simulink model "chap1_1sim"  (Simulink 8.1)
settings: Solver=ode45  StartTime=0.0  StopTime=20  RelTol=1e-3
settings Model: Creator=hp  LastModifiedBy=liujk
settings DataIOCC: SignalLoggingName=sigsOut
settings OptimizationCC: InitFltsAndDblsToZero=on
settings DebuggingCC: SaveWithParameterizedLinksMsg=none  SignalResolutionControl=TryResolveAllWithWarning  SolverPrmCheckMsg=none  MultiTaskDSMMsg=warning  MultiTaskCondExecSysMsg=none  StrictBusMsg=None
settings HardwareCC: TargetUnknown=on
settings RTWCC: IncludeERTFirstTime=on
settings GRTTargetCC: TargetFcnLib=ansi_tfl_tmw.mat

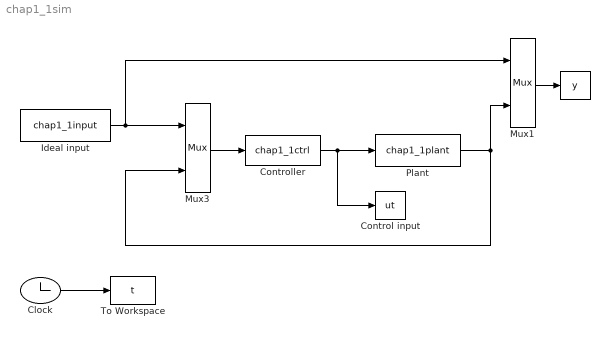
== system chap1_1sim ==
  " " : ToWorkspace  VariableName=y  SampleTime=-1
  Clock : Clock
  Control input : ToWorkspace  VariableName=ut  SampleTime=-1
  Controller : S-Function  FunctionName=chap1_1ctrl  EnableBusSupport=off
  Ideal input : S-Function  FunctionName=chap1_1input  EnableBusSupport=off
  Mux1 : Mux  Inputs=2
  Mux3 : Mux  Inputs=2
  Plant : S-Function  FunctionName=chap1_1plant  EnableBusSupport=off
  To Workspace : ToWorkspace  VariableName=t  SampleTime=-1
  wires:
  Controller/1 -> Control input/1, Plant/1
  Plant/1 -> Mux1/2, Mux3/2
  Mux1/1 -> " "/1
  Clock/1 -> To Workspace/1
  Mux3/1 -> Controller/1
  Ideal input/1 -> Mux1/1, Mux3/1
